simulink model "EX27"  (R2014a)
settings: Solver=FixedStepDiscrete  StartTime=0.0  StopTime=.5  FixedStep=7.629e-6  RelTol=1e-3
settings Model: Creator=Dennis Silage  LastModifiedBy=Silage
settings DataIOCC: SignalLoggingSaveFormat=ModelDataLogs
settings OptimizationCC: ExpressionDepthLimit=2147483647  InitFltsAndDblsToZero=on
settings DebuggingCC: UnderspecifiedInitializationDetection=Classic  FcnCallInpInsideContextMsg=UseLocalSettings  StateNameClashWarn=warning  StrictBusMsg=Warning
settings GRTTargetCC: CombineOutputUpdateFcns=off  GRTInterface=on

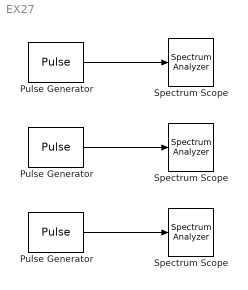
== system EX27 ==
  "Pulse Generator " : DiscretePulseGenerator  Period=65536  PulseWidth=32768  SampleTime=7.629e-6
  Pulse Generator : DiscretePulseGenerator  Period=65536  PulseWidth=8192  SampleTime=7.629e-6
  "Pulse Generator " : DiscretePulseGenerator  Period=65536  PulseWidth=16384  SampleTime=7.629e-6
  Spectrum Scope : SpectrumAnalyzer
  Spectrum Scope : SpectrumAnalyzer
  "Spectrum Scope " : SpectrumAnalyzer
  wires:
  Pulse Generator/1 -> Spectrum Scope/1
  "Pulse Generator "/1 -> "Spectrum Scope "/1
  "Pulse Generator "/1 -> Spectrum Scope/1
